simulink model "IlkOrnekBaranA"  (R2015a)
settings: Solver=ode45  StartTime=0.0  StopTime=inf  RelTol=1e-3
libraries: dspsrcs4 x2, dspsnks4 x1
settings Model: Creator=baran_000  LastModifiedBy=Baran

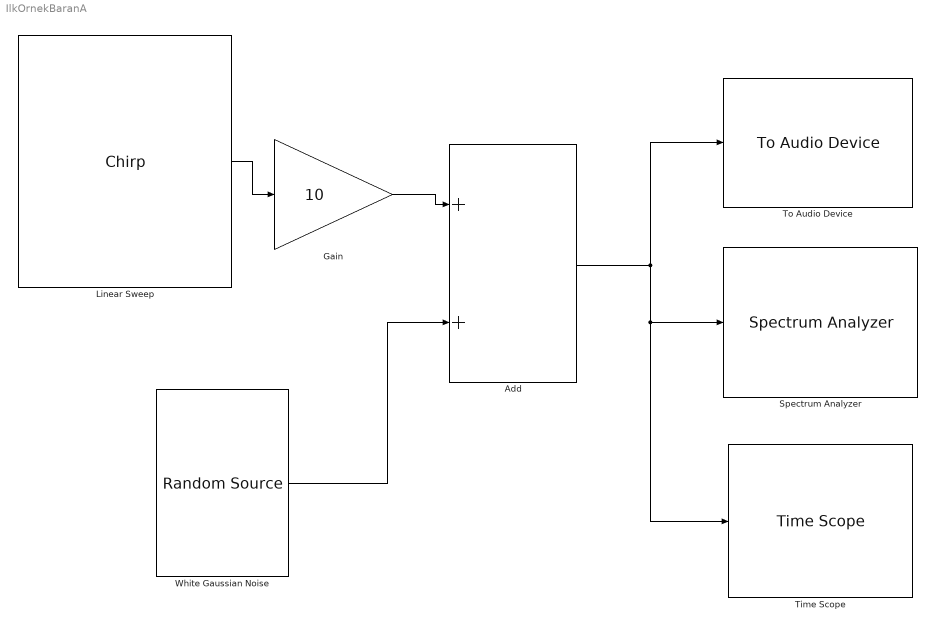
== system IlkOrnekBaranA ==
  Add : Sum
  Gain : Gain  Gain=10
  Linear Sweep : dspsrcs4/Chirp  sweep=Linear  mode=Bidirectional  f0=0  f1=1500  t1=1  Tsweep=1  phase=0  Ts=1/8000  spf=1024  datatype=Double
  Spectrum Analyzer : SpectrumAnalyzer
  Time Scope : TimeScope  DefaultConfigurationName=spbscopes.TimeScopeBlockCfg
  To Audio Device : dspsnks4/To Audio Device  deviceName=Default  inheritSampleRate=on  sampleRate=44100  deviceDatatype=Determine from input data type  autoBufferSize=on  bufferSize=4096  queueDuration=1.0  defaultOutputChannelMapping=on  outputChannelMapping=1:2  outputNumUnderrunSamples=off
  "White Gaussian Noise " : dspsrcs4/Random Source  SrcType=Gaussian  NormMethod=Ziggurat  CltLength=12  MinVal=0  MaxVal=1  MeanVal=0.1  VarVal=1  RepMode=Not repeatable  rawSeed=1  IsInherit=off  SampMode=Discrete  SampTime=1/8000  SampFrame=1024  DataType=Double  OutComplex=Real
  wires:
  "White Gaussian Noise "/1 -> Add/2
  Add/1 -> Time Scope/1, Spectrum Analyzer/1, To Audio Device/1
  Gain/1 -> Add/1
  Linear Sweep/1 -> Gain/1
